simulink model "fxpdemo_series_cascade_form"  (Simulink 7.6)
settings: Solver=FixedStepDiscrete  SolverMode=SingleTasking  StartTime=0.0  StopTime=200.0  FixedStep=1  RelTol=1e-3
Description:
  | Fixed-Point Series Cascade Form Filter
  | 
  | A fixed-point series cascade form filter can be constructed using the fundamental
  | building blocks of delay, sum, and gain.
settings Model: MinMaxOverflowLogging=MinMaxAndOverflow  Creator=The MathWorks Inc.  CovMetricSettings=d  ExtModeTrigMode=oneshot  ExtModeArmWhenConnect=off  ExtModeAutoUpdateStatusClock=off
settings DataIOCC: LimitDataPoints=off  SignalLoggingName=sigsOut
settings OptimizationCC: InlineParams=on  InitFltsAndDblsToZero=on
settings DebuggingCC: SaveWithParameterizedLinksMsg=none  SignalResolutionControl=TryResolveAllWithWarning  SolverPrmCheckMsg=none  MultiTaskDSMMsg=warning  MultiTaskCondExecSysMsg=none  IntegerOverflowMsg=none  ParameterDowncastMsg=warning  ParameterOverflowMsg=warning  ParameterPrecisionLossMsg=none  StrictBusMsg=None
settings HardwareCC: TargetUnknown=on
settings RTWCC: GenerateReport=on  IncludeERTFirstTime=on
settings GRTTargetCC: TargetFcnLib=ansi_tfl_tmw.mat

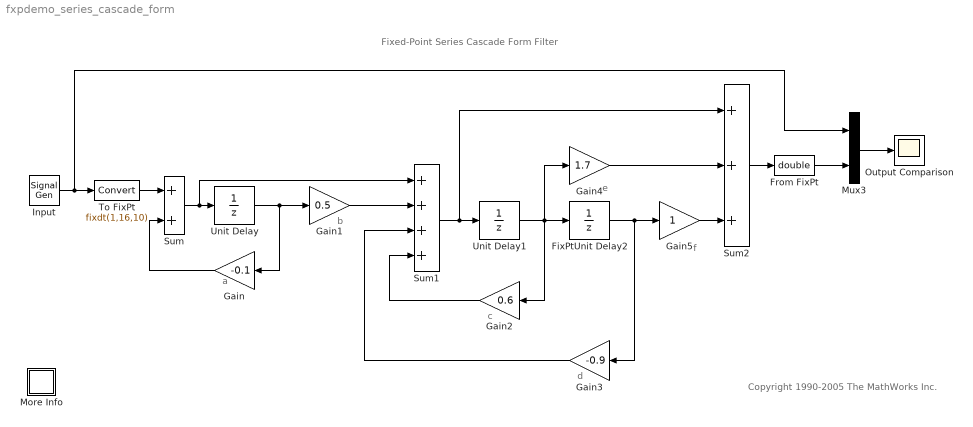
== system fxpdemo_series_cascade_form ==
  note: b
  note: c
  note: d
  note: f
  note: a
  note: e
  note: Copyright 1990-2005 The MathWorks Inc.
  note: Fixed-Point Series Cascade Form Filter
  " To FixPt" : DataTypeConversion  OutDataTypeStr=fixdt(1,16,10)
  FixPtUnit Delay2 : UnitDelay  X0=0.0  SampleTime=1.0
  From FixPt : DataTypeConversion  OutDataTypeStr=double
  Gain : Gain  Gain=-0.1  ParamDataTypeStr=sfix( 16 )  OutDataTypeStr=fixdt(1,16,10)
  Gain1 : Gain  Gain=0.5  ParamDataTypeStr=sfix( 16 )  OutDataTypeStr=fixdt(1,16,10)
  Gain2 : Gain  Gain=0.6  ParamDataTypeStr=sfix( 16 )  OutDataTypeStr=fixdt(1,16,10)
  Gain3 : Gain  Gain=-0.9  ParamDataTypeStr=sfix( 16 )  OutDataTypeStr=fixdt(1,16,10)
  Gain4 : Gain  Gain=1.7  ParamDataTypeStr=sfix( 16 )  OutDataTypeStr=fixdt(1,16,10)
  Gain5 : Gain  ParamDataTypeStr=sfix( 16 )  OutDataTypeStr=fixdt(1,16,10)
  Input : SignalGenerator  WaveForm=square  Frequency=0.005
  More Info : Subsystem
      settings: OpenFcn=showdemo(bdroot(gcs))
      mask Display: disp('?')
  Mux3 : Mux  Inputs=2
  Output Comparison : Scope
      settings: TickLabels=on  TimeRange=200  YMin=-8  YMax=10  SaveName=OutputComparison
  Sum : Sum  OutDataTypeStr=fixdt(1,16,10)
  Sum1 : Sum  Inputs=++++  OutDataTypeStr=fixdt(1,16,10)
  Sum2 : Sum  Inputs=+++  OutDataTypeStr=fixdt(1,16,10)
  Unit Delay : UnitDelay  X0=0.0  SampleTime=1.0
  Unit Delay1 : UnitDelay  X0=0.0  SampleTime=1.0
  wires:
  " To FixPt"/1 -> Sum/1
  Input/1 -> " To FixPt"/1, Mux3/1
  Gain/1 -> Sum/2
  Sum/1 -> Unit Delay/1, Sum1/1
  Unit Delay/1 -> Gain1/1, Gain/1
  Gain1/1 -> Sum1/2
  Gain2/1 -> Sum1/4
  Sum1/1 -> Unit Delay1/1, Sum2/1
  Unit Delay1/1 -> FixPtUnit Delay2/1, Gain2/1, Gain4/1
  Gain3/1 -> Sum1/3
  FixPtUnit Delay2/1 -> Gain3/1, Gain5/1
  Gain5/1 -> Sum2/3
  Gain4/1 -> Sum2/2
  Sum2/1 -> From FixPt/1
  From FixPt/1 -> Mux3/2
  Mux3/1 -> Output Comparison/1

== system fxpdemo_series_cascade_form/More Info ==
